simulink model "ACS_AP"  (R2022b)
settings: Solver=ode1  StartTime=0.0  StopTime=200  FixedStep=0.05  RelTol=1e-3  EnableMultiTasking=on
undefined symbols (not defined in the file): ACSP
settings Model: Creator=jmbianni  LastModifiedBy=bendr
settings SolverCC: AlgebraicLoopSolver=TrustRegion
settings DataIOCC: InitialState=[]  LimitDataPoints=on  LoadInitialState=on  SaveFormat=Array  ReturnWorkspaceOutputs=off
settings OptimizationCC: DefaultParameterBehavior=Inlined  BufferReuse=off  ExpressionDepthLimit=2147483647  LifeSpan=inf
settings DebuggingCC: ArtificialAlgebraicLoopMsg=none  UnderspecifiedInitializationDetection=Classic  MergeDetectMultiDrivingBlocksExec=none  UnconnectedInputMsg=warning  UnconnectedOutputMsg=warning  UnconnectedLineMsg=warning  StateNameClashWarn=warning  InitInArrayFormatMsg=none  SFUnexpectedBacktrackingDiag=warning  SFNoUnconditionalDefaultTransitionDiag=warning  SFExecutionAtInitializationDiag=none  SFMachineParentedDataDiag=warning  ArithmeticOperatorsInVariantConditions=warning
settings HardwareCC: ProdBitPerPointer=32  ProdBitPerSizeT=32  ProdBitPerPtrDiffT=32  ProdLargestAtomicFloat=None  ProdIntDivRoundTo=Undefined  ProdEndianess=Unspecified  ProdWordSize=32  ProdHWDeviceType=32-bit Generic
settings ModelReferenceCC: PropagateSignalLabelsOutOfModel=off
settings SFSimCC: SimUseLocalCustomCode=off  CustomCodeUndefinedFunction=UseInterfaceOnly
settings RTWCC: RTWUseLocalCustomCode=off
settings CodeAppCC: StateflowObjectComments=on
settings GRTTargetCC: TargetLangStandard=C89/C90 (ANSI)
settings ConfigComp: CovMetricSettings=dw  CovSaveCumulativeToWorkspaceVar=on  CovSaveSingleToWorkspaceVar=on  CovExternalEMLEnable=off

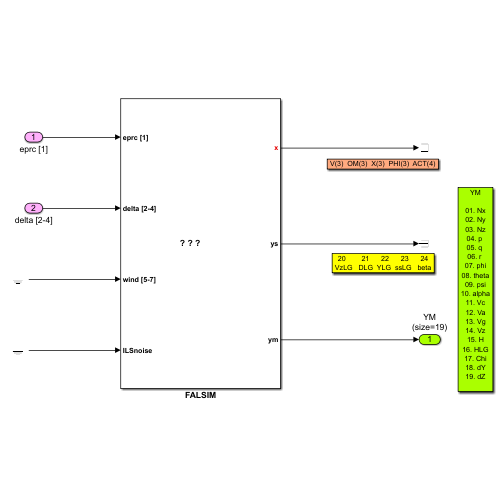
[thumbnail: Simulink's stored preview of the top-level diagram]
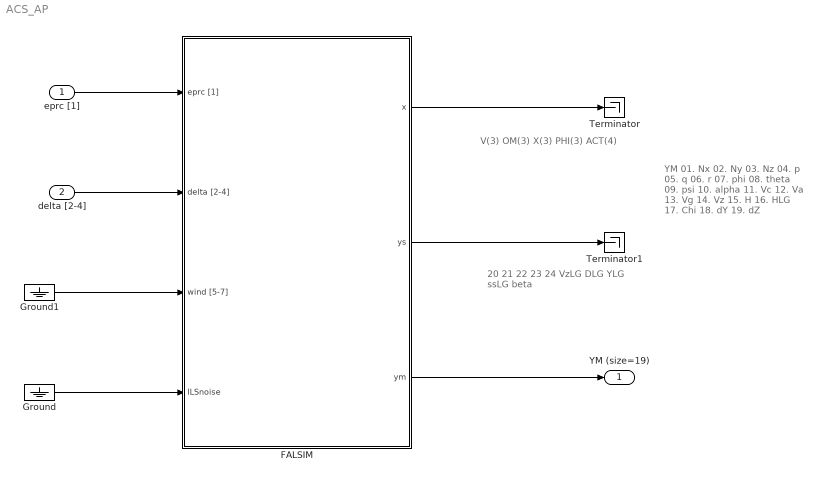
== system ACS_AP ==
  note: 20        21      22      23      24
      | VzLG   DLG  YLG  ssLG   beta
  note: YM
      |
      | 01. Nx
      | 02. Ny
      | 03. Nz
      | 04. p
      | 05. q
      | 06. r
      | 07. phi
      | 08. theta
      | 09. psi
      | 10. alpha
      | 11. Vc
      | 12. Va
      | 13. Vg
      | 14. Vz
      | 15. H
      | 16. HLG
      | 17. Chi
      | 18. dY
      | 19. dZ
  note: V(3) OM(3) X(3) PHI(3) ACT(4)
  eprc [1] : Inport
  delta [2-4] : Inport  Port=2  PortDimensions=3
  FALSIM : Subsystem
      mask Display:
      | image(imread('FALSIM.png'));
      | color('white');
      | 
      | color('red');
      | disp('http://w3.onera.fr/smac/ \n\n\n\n');
      | 
      | 
      | 
      | color('red');
      | %disp('{\bf\fontsize{12}SMAC TOOLS}', 'texmode','on');
      | 
      | color('yellow');
      | 
      | port_label('output', 1,'{\bf\fontsize{12}States}', 'texmode','on');
      | port_label('output', 2,'{\bf\fontsize{12}Non Measured Outputs}', 'texmode','on');
      | port_label('output', 3,'{\bf\fontsize{12}Measured Outputs}', 'texmode','on');
      | port_label('input', 1,'{\bf\fontsize{12}\delta_{TH}}', 'texmode','on');
      | port_label('input', 2,'{\bf\fontsize{12}\delta_A , \delta_E , \delta_R}', 'texmode','on');
      | port_label('input', 3,'{\bf\fontsize{12}W_x , W_y , W_z}', 'texmode','on');
      | port_label('input', 4,'{\bf\fontsize{12}W_{LOC} , W_{GLD}}', 'texmode','on');
  Ground : Ground
  Ground1 : Ground
  Terminator : Terminator
  Terminator1 : Terminator
  YM (size=19) : Outport
  wires:
  FALSIM/1(x) -> Terminator/1
  eprc [1]/1 -> FALSIM/1(eprc [1])
  delta [2-4]/1 -> FALSIM/2(delta [2-4])
  FALSIM/2(ys) -> Terminator1/1
  Ground/1 -> FALSIM/4(ILSnoise)
  Ground1/1 -> FALSIM/3(wind [5-7])
  FALSIM/3(ym) -> YM (size=19)/1

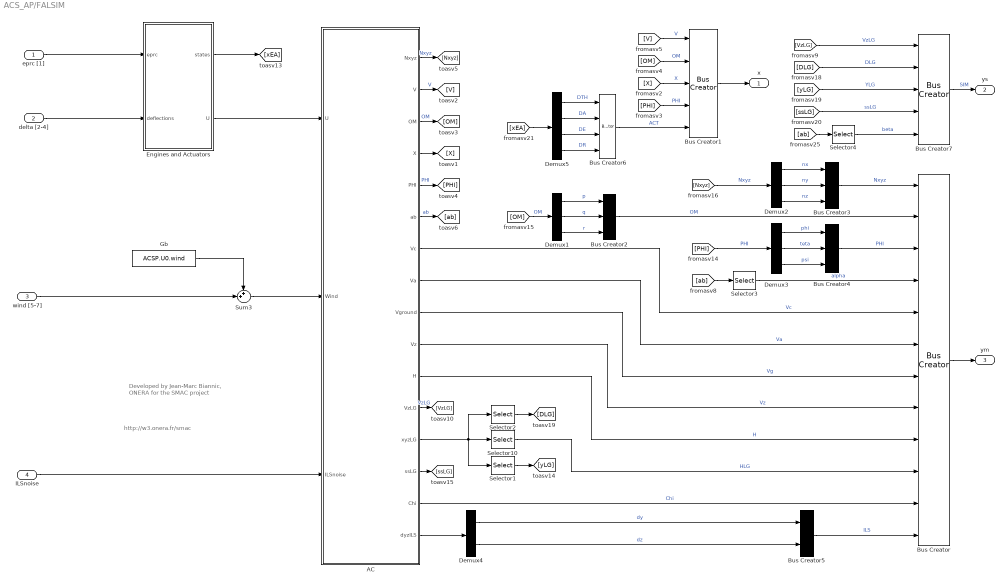
== system ACS_AP/FALSIM ==
  note: Developed by
      | Jean-Marc Biannic, ONERA
      | for the SMAC project
  note: http://w3.onera.fr/smac
  eprc [1] : Inport
  delta [2-4] : Inport  Port=2  PortDimensions=3
  wind [5-7] : Inport  Port=3  PortDimensions=3
  ILSnoise : Inport  Port=4  PortDimensions=2
  AC : Subsystem
  Bus Creator : BusCreator  Inputs=12
  Bus Creator1 : BusCreator  Inputs=5
  Bus Creator2 : BusCreator  Inputs=3
  Bus Creator3 : BusCreator  Inputs=3
  Bus Creator4 : BusCreator  Inputs=3
  Bus Creator5 : BusCreator  Inputs=2
  Bus Creator6 : BusCreator  Inputs=4
  Bus Creator7 : BusCreator  Inputs=5
  Demux1 : Demux  Outputs=3
  Demux2 : Demux  Outputs=3
  Demux3 : Demux  Outputs=3
  Demux4 : Demux  Outputs=2
  Demux5 : Demux
  Engines and Actuators : Subsystem
  Gb : Constant  Value=ACSP.U0.wind
  Selector1 : Selector  InputPortWidth=3  IndexOptions=Index vector (dialog)  Indices=2  OutputSizes=1
  Selector10 : Selector  InputPortWidth=3  IndexOptions=Index vector (dialog)  Indices=3  OutputSizes=1
  Selector2 : Selector  InputPortWidth=3  IndexOptions=Index vector (dialog)  Indices=1  OutputSizes=1
  Selector3 : Selector  InputPortWidth=2  IndexOptions=Index vector (dialog)  Indices=1  OutputSizes=1
  Selector4 : Selector  InputPortWidth=2  IndexOptions=Index vector (dialog)  Indices=2  OutputSizes=1
  Sum3 : Sum  Inputs=++|
  x : Outport
  ys : Outport  Port=2
  ym : Outport  Port=3
  wires:
  wind [5-7]/1 -> Sum3/2
  Selector3/1 -> Bus Creator/4  "alpha"
  [ab] -> Selector3/1
  Bus Creator2/1 -> Bus Creator/2  "OM"
  Demux1/3 -> Bus Creator2/3  "r"
  Demux1/2 -> Bus Creator2/2  "q"
  Demux1/1 -> Bus Creator2/1  "p"
  [OM] -> Demux1/1  "OM"
  Demux2/3 -> Bus Creator3/3  "nz"
  Demux2/2 -> Bus Creator3/2  "ny"
  Demux2/1 -> Bus Creator3/1  "nx"
  [Nxyz] -> Demux2/1  "Nxyz"
  Bus Creator3/1 -> Bus Creator/1  "Nxyz"
  Demux3/3 -> Bus Creator4/3  "psi"
  Demux3/2 -> Bus Creator4/2  "teta"
  Demux3/1 -> Bus Creator4/1  "phi"
  [PHI] -> Demux3/1  "PHI"
  Bus Creator4/1 -> Bus Creator/3  "PHI"
  AC/13(xyzLG) -> Selector1/1, Selector10/1, Selector2/1
  Selector1/1 -> [yLG]
  AC/14(ssLG) -> [ssLG]
  AC/16(dyzILS) -> Demux4/1
  Demux4/1 -> Bus Creator5/1  "dy"
  Demux4/2 -> Bus Creator5/2  "dz"
  Selector2/1 -> [DLG]
  Selector10/1 -> Bus Creator/10  "HLG"
  AC/1(Nxyz) -> [Nxyz]  "Nxyz"
  AC/2(V) -> [V]  "V"
  AC/3(OM) -> [OM]  "OM"
  AC/4(X) -> [X]
  AC/5(PHI) -> [PHI]  "PHI"
  AC/6(ab) -> [ab]  "ab"
  AC/7(Vc) -> Bus Creator/5  "Vc"
  AC/8(Va) -> Bus Creator/6  "Va"
  AC/9(Vground) -> Bus Creator/7  "Vg"
  AC/15(Chi) -> Bus Creator/11  "Chi"
  AC/12(VzLG) -> [VzLG]  "VzLG"
  [V] -> Bus Creator1/1  "V"
  [OM] -> Bus Creator1/2  "OM"
  [X] -> Bus Creator1/3  "X"
  [PHI] -> Bus Creator1/4  "PHI"
  Bus Creator1/1 -> x/1
  eprc [1]/1 -> Engines and Actuators/1(eprc)
  Engines and Actuators/2(U) -> AC/1(U)
  Engines and Actuators/1(states) -> [xEA]
  Demux5/1 -> Bus Creator6/1  "DTH"
  Demux5/2 -> Bus Creator6/2  "DA"
  Demux5/3 -> Bus Creator6/3  "DE"
  Demux5/4 -> Bus Creator6/4  "DR"
  [xEA] -> Demux5/1
  Bus Creator6/1 -> Bus Creator1/5  "ACT"
  Bus Creator5/1 -> Bus Creator/12  "ILS"
  [ab] -> Selector4/1
  AC/10(Vz) -> Bus Creator/8  "Vz"
  AC/11(H) -> Bus Creator/9  "H"
  ILSnoise/1 -> AC/3(ILSnoise)
  Gb/1 -> Sum3/1
  Sum3/1 -> AC/2(Wind)
  Bus Creator/1 -> ym/1
  Bus Creator7/1 -> ys/1  "SIM"
  delta [2-4]/1 -> Engines and Actuators/2(deflections)
  Selector4/1 -> Bus Creator7/5  "beta"
  [ssLG] -> Bus Creator7/4  "ssLG"
  [yLG] -> Bus Creator7/3  "YLG"
  [DLG] -> Bus Creator7/2  "DLG"
  [VzLG] -> Bus Creator7/1  "VzLG"

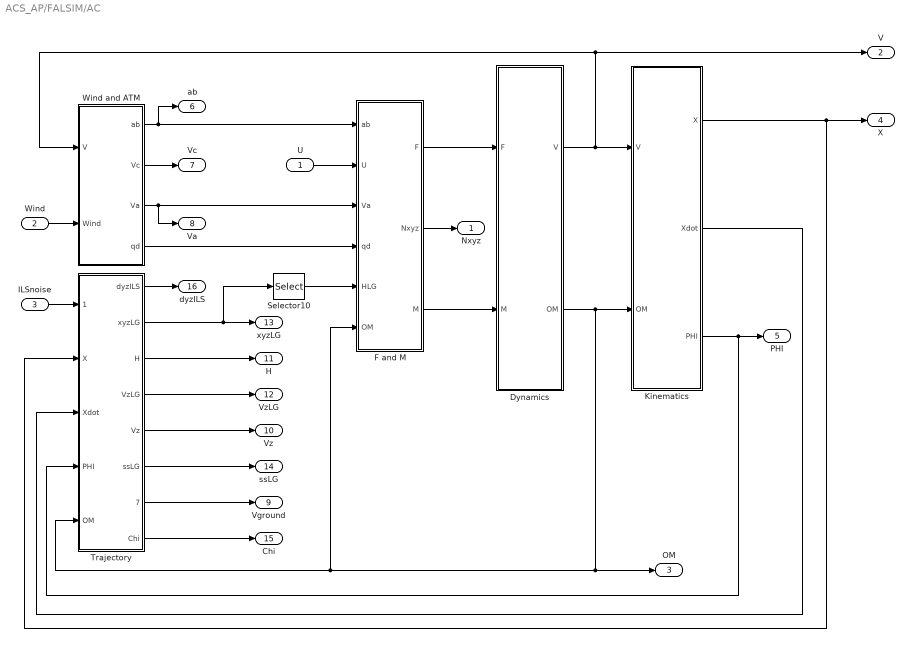
== system ACS_AP/FALSIM/AC ==
  U : Inport
  Wind : Inport  Port=2  PortDimensions=3
  ILSnoise : Inport  Port=3  PortDimensions=2
  Dynamics : Subsystem
  F and M : Subsystem
  Kinematics : Subsystem
  Selector10 : Selector  InputPortWidth=3  IndexOptions=Index vector (dialog)  Indices=3  OutputSizes=1
  Trajectory : Subsystem
  Wind and ATM : Subsystem
  Nxyz : Outport
  V : Outport  Port=2
  OM : Outport  Port=3
  X : Outport  Port=4
  PHI : Outport  Port=5
  ab : Outport  Port=6
  Vc : Outport  Port=7
  Va : Outport  Port=8
  Vground : Outport  Port=9
  Vz : Outport  Port=10
  H : Outport  Port=11
  VzLG : Outport  Port=12
  xyzLG : Outport  Port=13
  ssLG : Outport  Port=14
  Chi : Outport  Port=15
  dyzILS : Outport  Port=16
  wires:
  F and M/2(Nxyz) -> Nxyz/1
  Wind and ATM/1(ab) -> F and M/1(ab), ab/1
  U/1 -> F and M/2(U)
  Wind and ATM/4(qd) -> F and M/4(qd)
  Wind and ATM/3(Va) -> F and M/3(Va), Va/1
  Wind and ATM/2(Vc) -> Vc/1
  Wind/1 -> Wind and ATM/2(Wind)
  Kinematics/2(Xdot) -> Trajectory/3(Xdot)
  Kinematics/3(PHI) -> Trajectory/4(PHI), PHI/1
  Dynamics/2(OM) -> Kinematics/2(OM), OM/1, F and M/6(OM), Trajectory/5(OM)
  Dynamics/1(V) -> Kinematics/1(V), V/1, Wind and ATM/1(V)
  F and M/1(F) -> Dynamics/1(F)
  F and M/3(M) -> Dynamics/2(M)
  Kinematics/1(X) -> X/1, Trajectory/2(X)
  Selector10/1 -> F and M/5(HLG)
  Trajectory/2(xyzLG) -> xyzLG/1, Selector10/1
  Trajectory/1(dyzILS) -> dyzILS/1
  Trajectory/4(VzLG) -> VzLG/1
  Trajectory/8(Chi) -> Chi/1
  Trajectory/7(Vground) -> Vground/1
  Trajectory/6(ssLG) -> ssLG/1
  Trajectory/3(H) -> H/1
  Trajectory/5(Vz) -> Vz/1
  ILSnoise/1 -> Trajectory/1(ILSnoise)

== system ACS_AP/FALSIM/Engines and Actuators ==
  eprc : Inport
  deflections : Inport  Port=2
  Actuators : Subsystem
  Engines : Subsystem
  Mux : Mux  Inputs=2
  Mux1 : Mux  Inputs=2
  Sum3 : Sum  Inputs=|++
  delta0 : Constant  Value=ACSP.U0.delta
  epr0 : Constant  Value=ACSP.U0.epr
  states : Outport
  U : Outport  Port=2
  wires:
  Actuators/1(delta) -> Sum3/1, Mux1/2
  Engines/1(TH) -> Mux/1
  eprc/1 -> Engines/2(eprc)
  deflections/1 -> Actuators/1(deltac)
  epr0/1 -> Engines/1(epr0)
  Mux/1 -> U/1
  Engines/2(epr) -> Mux1/1  "EPR"
  Mux1/1 -> states/1
  Sum3/1 -> Mux/2
  delta0/1 -> Sum3/2

== system ACS_AP/FALSIM/AC/Dynamics ==
  note: F =mass*(Vdot + OM x V)
  note: M = I*OMdot + OM x (I*OM)
  F : Inport
  M : Inport  Port=2
  CP1 : Subsystem
      mask Display:
      | fprintf('CROSS \n PRODUCT');
      | color('red');
      | fprintf('\n\n');
      | fprintf(' \n \n \n z=x^y');
      | %text(3,1,'PRODUCT');
      | %text(5,1,'z=x^y');
  CP2 : Subsystem
      mask Display:
      | fprintf('CROSS \n PRODUCT');
      | color('red');
      | fprintf('\n\n');
      | fprintf(' \n \n \n z=x^y');
      | %text(3,1,'PRODUCT');
      | %text(5,1,'z=x^y');
  Inertia : Gain  Gain=reshape(ACSP.MIG.I,3,3)  Multiplication=Matrix(K*u)
  Inertia^-1 : Gain  Gain=ACSP.MIG.J  Multiplication=Matrix(K*u)
  Int_OM : Integrator  InitialCondition=ACSP.X0.OM  ContinuousStateAttributes='OM'
  Int_V : Integrator  InitialCondition=ACSP.X0.V  ContinuousStateAttributes='V'
  Mass^-1 : Gain  Gain=1/ACSP.MIG.mass
  Sum : Sum  Inputs=|+-
  Sum1 : Sum  Inputs=-+|
  V : Outport
  OM : Outport  Port=2
  wires:
  Int_V/1 -> CP2/2(y), V/1
  Sum1/1 -> Int_V/1
  Sum/1 -> Inertia^-1/1
  M/1 -> Sum/1
  Inertia^-1/1 -> Int_OM/1
  F/1 -> Mass^-1/1
  Int_OM/1 -> CP1/1(x), Inertia/1, CP2/1(x), OM/1
  CP2/1(z) -> Sum1/1
  CP1/1(z) -> Sum/2
  Mass^-1/1 -> Sum1/2
  Inertia/1 -> CP1/2(y)

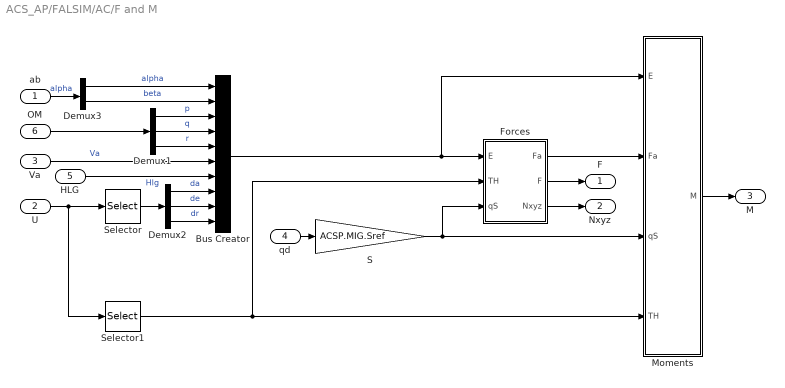
== system ACS_AP/FALSIM/AC/F and M ==
  ab : Inport
  U : Inport  Port=2
  Va : Inport  Port=3
  qd : Inport  Port=4
  HLG : Inport  Port=5
  OM : Inport  Port=6
  Bus Creator : BusCreator  Inputs=10
  Demux1 : Demux  Outputs=3
  Demux2 : Demux  Outputs=3
  Demux3 : Demux  Outputs=2
  Forces : Subsystem
  Moments : Subsystem
  S : Gain  Gain=ACSP.MIG.Sref
  Selector : Selector  InputPortWidth=4  IndexOptions=Index vector (dialog)  Indices=[2 3 4]  OutputSizes=1
  Selector1 : Selector  InputPortWidth=4  IndexOptions=Index vector (dialog)  Indices=[1]  OutputSizes=1
  F : Outport
  Nxyz : Outport  Port=2
  M : Outport  Port=3
  wires:
  Forces/3(Nxyz) -> Nxyz/1
  Selector1/1 -> Moments/4(TH), Forces/2(TH)
  Forces/2(F) -> F/1
  S/1 -> Moments/3(qS), Forces/3(qS)
  Forces/1(Fa) -> Moments/2(Fa)
  U/1 -> Selector/1, Selector1/1
  Selector/1 -> Demux2/1
  Moments/1(M) -> M/1
  Bus Creator/1 -> Moments/1(E), Forces/1(E)
  Demux1/1 -> Bus Creator/3  "p"
  Demux1/2 -> Bus Creator/4  "q"
  Demux1/3 -> Bus Creator/5  "r"
  Demux3/2 -> Bus Creator/2  "beta"
  Demux2/3 -> Bus Creator/10  "dr"
  Demux2/2 -> Bus Creator/9  "de"
  Demux2/1 -> Bus Creator/8  "da"
  Va/1 -> Bus Creator/6  "Va"
  HLG/1 -> Bus Creator/7  "Hlg"
  OM/1 -> Demux1/1
  qd/1 -> S/1
  Demux3/1 -> Bus Creator/1  "alpha"
  ab/1 -> Demux3/1  "alpha"

== system ACS_AP/FALSIM/AC/Kinematics ==
  V : Inport
  OM : Inport  Port=2
  Int_PHI : Integrator  InitialCondition=ACSP.X0.PHI  ContinuousStateAttributes='PHI'
  Int_X : Integrator  InitialCondition=ACSP.X0.X  ContinuousStateAttributes='X'
  R(PHI) : Subsystem
      mask Display:
      | fprintf('MATRIX \n PRODUCT');
      | color('red');
      | fprintf('\n\n');
      | fprintf(' \n \n \n z=M(x)*y');
  Rotations and transformations matrices : Subsystem
  T(PHI) : Subsystem
      mask Display:
      | fprintf('MATRIX \n PRODUCT');
      | color('red');
      | fprintf('\n\n');
      | fprintf(' \n \n \n z=M(x)*y');
  X : Outport
  Xdot : Outport  Port=2
  PHI : Outport  Port=3
  tag scope: RV2B=global
  wires:
  T(PHI)/1(z) -> Int_PHI/1
  Rotations and transformations matrices/2(RV2B) -> [RV2B]
  Rotations and transformations matrices/1(TPHI) -> T(PHI)/1(x)
  Rotations and transformations matrices/3(RB2V) -> R(PHI)/1(x)
  Int_X/1 -> X/1
  Int_PHI/1 -> PHI/1, Rotations and transformations matrices/1(PHI)
  R(PHI)/1(z) -> Xdot/1, Int_X/1
  V/1 -> R(PHI)/2(y)
  OM/1 -> T(PHI)/2(y)

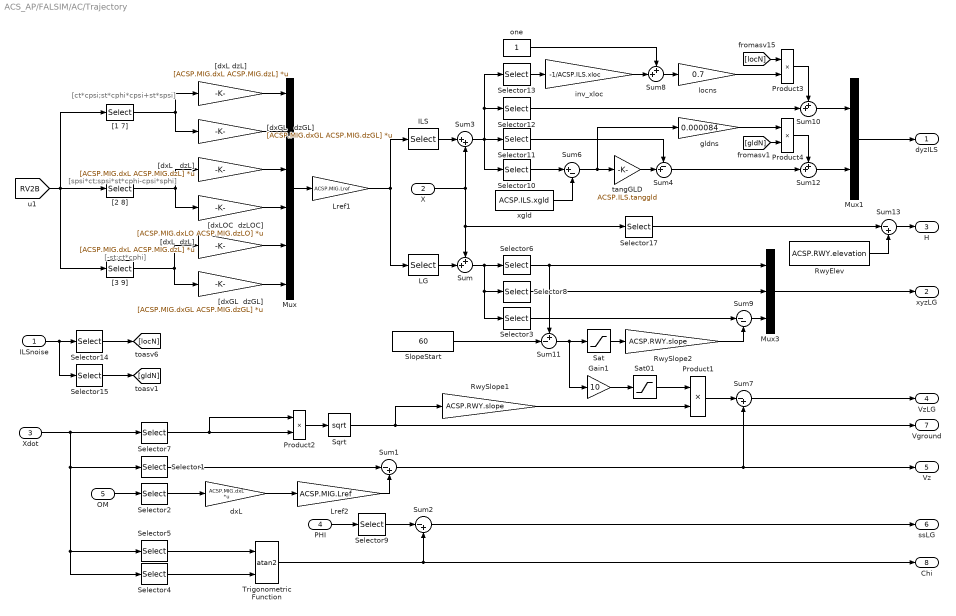
== system ACS_AP/FALSIM/AC/Trajectory ==
  note: [-st;ct*cphi]
  note: [ct*cpsi;st*cphi*cpsi+st*spsi]
  note: [spsi*ct;spsi*st*cphi-cpsi*sphi]
  ILSnoise : Inport
  X : Inport  Port=2
  Xdot : Inport  Port=3
  PHI : Inport  Port=4
  OM : Inport  Port=5
  Gain1 : Gain  Gain=10
  ILS : Selector  InputPortWidth=6  IndexOptions=Index vector (dialog)  Indices=[2 4 6]  OutputSizes=1
  LG : Selector  InputPortWidth=6  IndexOptions=Index vector (dialog)  Indices=[1 3 5]  OutputSizes=1
  Lref1 : Gain  Gain=ACSP.MIG.Lref
  Lref2 : Gain  Gain=ACSP.MIG.Lref
  Mux : Mux  Inputs=6
  Mux1 : Mux  Inputs=2
  Mux3 : Mux  Inputs=3
  Product{1..4} (4 alike) : Product  InputSameDT=on  RndMeth=Zero  SaturateOnIntegerOverflow=on  OutDataTypeStr=Inherit: Same as first input
  RwyElev : Constant  Value=ACSP.RWY.elevation
  RwySlope1 : Gain  Gain=ACSP.RWY.slope
  RwySlope2 : Gain  Gain=ACSP.RWY.slope
  Sat : Saturate  UpperLimit=1000  LowerLimit=0
  Sat01 : Saturate  UpperLimit=1  LowerLimit=0
  Selector{1,3,9,11,17} (5 alike) : Selector  InputPortWidth=3  IndexOptions=Index vector (dialog)  Indices=3  OutputSizes=1
  Selector{4,6..7,10,13} (5 alike) : Selector  InputPortWidth=3  IndexOptions=Index vector (dialog)  Indices=1  OutputSizes=1
  Selector{2,5,8,12} (4 alike) : Selector  InputPortWidth=3  IndexOptions=Index vector (dialog)  Indices=2  OutputSizes=1
  Selector14 : Selector  InputPortWidth=2  IndexOptions=Index vector (dialog)  Indices=1  OutputSizes=1
  Selector15 : Selector  InputPortWidth=2  IndexOptions=Index vector (dialog)  Indices=2  OutputSizes=1
  SlopeStart : Constant  Value=60
  Sqrt : Sqrt
  Sum{,8,10,12} (4 alike) : Sum  Inputs=++|
  Sum{1..2,7,13} (4 alike) : Sum  Inputs=|-+
  Sum11 : Sum  Inputs=+-|
  Sum3 : Sum  Inputs=|++
  Sum4 : Sum  Inputs=-+|
  Sum6 : Sum  Inputs=|+-
  Sum9 : Sum  Inputs=|--
  Trigonometric Function : Trigonometry  Operator=atan2
  "[1 7]" : Selector  InputPortWidth=9  IndexOptions=Index vector (dialog)  Indices=[1 7]  OutputSizes=1
  "[2 8]" : Selector  InputPortWidth=9  IndexOptions=Index vector (dialog)  Indices=[2 8]  OutputSizes=1
  "[3 9]" : Selector  InputPortWidth=9  IndexOptions=Index vector (dialog)  Indices=[3 9]  OutputSizes=1
  "[dxGL   dzGL]" : Gain  Gain=[ACSP.MIG.dxGL ACSP.MIG.dzGL]  Multiplication=Matrix(K*u)
  "[dxGL  dzGL]" : Gain  Gain=[ACSP.MIG.dxGL ACSP.MIG.dzGL]  Multiplication=Matrix(K*u)
  "[dxL   dzL]" : Gain  Gain=[ACSP.MIG.dxL ACSP.MIG.dzL]  Multiplication=Matrix(K*u)
  "[dxL  dzL]" : Gain  Gain=[ACSP.MIG.dxL ACSP.MIG.dzL]  Multiplication=Matrix(K*u)
  "[dxL dzL]" : Gain  Gain=[ACSP.MIG.dxL ACSP.MIG.dzL]  Multiplication=Matrix(K*u)
  "[dxLOC  dzLOC]" : Gain  Gain=[ACSP.MIG.dxLO ACSP.MIG.dzLO]  Multiplication=Matrix(K*u)
  dxL : Gain  Gain=ACSP.MIG.dxL  Multiplication=Matrix(K*u)
  gldns : Gain  Gain=0.000084
  inv_xloc : Gain  Gain=-1/ACSP.ILS.xloc
  locns : Gain  Gain=0.7
  one : Constant
  tangGLD : Gain  Gain=ACSP.ILS.tanggld
  xgld : Constant  Value=ACSP.ILS.xgld
  dyzILS : Outport
  xyzLG : Outport  Port=2
  H : Outport  Port=3
  VzLG : Outport  Port=4
  Vz : Outport  Port=5
  ssLG : Outport  Port=6
  Vground : Outport  Port=7
  Chi : Outport  Port=8
  wires:
  Xdot/1 -> Selector1/1, Selector4/1, Selector5/1, Selector7/1
  OM/1 -> Selector2/1
  Selector2/1 -> dxL/1
  dxL/1 -> Lref2/1
  Lref2/1 -> Sum1/2
  Sum1/1 -> Vz/1, Sum7/2
  [RV2B] -> "[1 7]"/1, "[3 9]"/1, "[2 8]"/1
  Selector1/1 -> Sum1/1
  Selector5/1 -> Trigonometric Function/1
  Trigonometric Function/1 -> Sum2/2, Chi/1
  "[1 7]"/1 -> "[dxL dzL]"/1, "[dxGL   dzGL]"/1
  Product2/1 -> Sqrt/1
  Selector4/1 -> Trigonometric Function/2
  Selector7/1 -> Product2/2, Product2/1
  Sqrt/1 -> Vground/1, RwySlope1/1
  "[2 8]"/1 -> "[dxL   dzL]"/1, "[dxLOC  dzLOC]"/1
  PHI/1 -> Selector9/1
  Selector9/1 -> Sum2/1
  Sum2/1 -> ssLG/1
  "[3 9]"/1 -> "[dxL  dzL]"/1, "[dxGL  dzGL]"/1
  "[dxL dzL]"/1 -> Mux/1
  "[dxGL   dzGL]"/1 -> Mux/2
  "[dxL   dzL]"/1 -> Mux/3
  "[dxLOC  dzLOC]"/1 -> Mux/4
  "[dxL  dzL]"/1 -> Mux/5
  "[dxGL  dzGL]"/1 -> Mux/6
  Mux/1 -> Lref1/1
  Lref1/1 -> LG/1, ILS/1
  ILS/1 -> Sum3/1
  Sum3/1 -> Selector10/1, Selector11/1, Selector12/1, Selector13/1
  Sum6/1 -> gldns/1, tangGLD/1
  Selector10/1 -> Sum6/1
  xgld/1 -> Sum6/2
  Mux1/1 -> dyzILS/1
  Selector12/1 -> Sum10/2
  Selector11/1 -> Sum4/1
  tangGLD/1 -> Sum4/2
  Sum4/1 -> Sum12/2
  LG/1 -> Sum/2
  X/1 -> Selector17/1, Sum/1, Sum3/2
  Sum/1 -> Selector6/1, Selector3/1, Selector8/1
  Sat01/1 -> Product1/1
  RwySlope1/1 -> Product1/2
  Sum11/1 -> Gain1/1, Sat/1
  Product1/1 -> Sum7/1
  Sat/1 -> RwySlope2/1
  Mux3/1 -> xyzLG/1
  Selector8/1 -> Mux3/2
  Selector6/1 -> Sum11/1, Mux3/1
  SlopeStart/1 -> Sum11/2
  Sum7/1 -> VzLG/1
  Gain1/1 -> Sat01/1
  Selector13/1 -> inv_xloc/1
  inv_xloc/1 -> Sum8/2
  one/1 -> Sum8/1
  Sum8/1 -> locns/1
  Sum10/1 -> Mux1/1
  locns/1 -> Product3/2
  Product3/1 -> Sum10/1
  Sum12/1 -> Mux1/2
  Product4/1 -> Sum12/1
  gldns/1 -> Product4/1
  ILSnoise/1 -> Selector15/1, Selector14/1
  Selector14/1 -> [locN]
  Selector15/1 -> [gldN]
  [locN] -> Product3/1
  [gldN] -> Product4/2
  RwyElev/1 -> Sum13/2
  Sum13/1 -> H/1
  Selector17/1 -> Sum13/1
  Sum9/1 -> Mux3/3
  RwySlope2/1 -> Sum9/2
  Selector3/1 -> Sum9/1

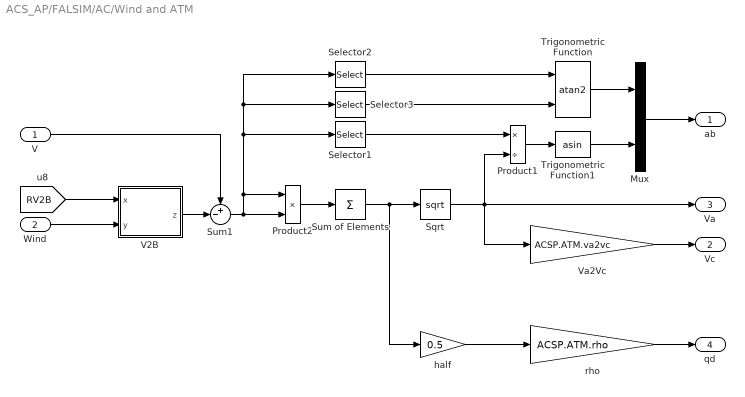
== system ACS_AP/FALSIM/AC/Wind and ATM ==
  V : Inport
  Wind : Inport  Port=2
  Mux : Mux  Inputs=2
  Product1 : Product  Inputs=*/  InputSameDT=on  RndMeth=Zero  SaturateOnIntegerOverflow=on  OutDataTypeStr=Inherit: Same as first input
  Product2 : Product  InputSameDT=on  RndMeth=Zero  SaturateOnIntegerOverflow=on  OutDataTypeStr=Inherit: Same as first input
  Selector1 : Selector  InputPortWidth=3  IndexOptions=Index vector (dialog)  Indices=2  OutputSizes=1
  Selector2 : Selector  InputPortWidth=3  IndexOptions=Index vector (dialog)  Indices=3  OutputSizes=1
  Selector3 : Selector  InputPortWidth=3  IndexOptions=Index vector (dialog)  Indices=1  OutputSizes=1
  Sqrt : Sqrt
  Sum of Elements : Sum  Inputs=+
  Sum1 : Sum  Inputs=+-|
  Trigonometric Function : Trigonometry  Operator=atan2
  Trigonometric Function1 : Trigonometry  Operator=asin
  V2B : Subsystem
      mask Display:
      | fprintf('MATRIX \n PRODUCT');
      | color('red');
      | fprintf('\n\n');
      | fprintf(' \n \n \n z=M(x)*y');
  Va2Vc : Gain  Gain=ACSP.ATM.va2vc
  half : Gain  Gain=0.5  SaturateOnIntegerOverflow=on  OutDataTypeStr=Inherit: Same as input  ParamDataTypeStr=Inherit: Same as input
  rho : Gain  Gain=ACSP.ATM.rho
  ab : Outport
  Vc : Outport  Port=2
  Va : Outport  Port=3
  qd : Outport  Port=4
  wires:
  Wind/1 -> V2B/2(y)
  rho/1 -> qd/1
  half/1 -> rho/1
  Va2Vc/1 -> Vc/1
  Sum1/1 -> Product2/2, Product2/1, Selector3/1, Selector2/1, Selector1/1
  Selector1/1 -> Product1/1
  Selector2/1 -> Trigonometric Function/1
  Selector3/1 -> Trigonometric Function/2
  [RV2B] -> V2B/1(x)
  V2B/1(z) -> Sum1/2
  V/1 -> Sum1/1
  Product2/1 -> Sum of Elements/1
  Sqrt/1 -> Va/1, Product1/2, Va2Vc/1
  Product1/1 -> Trigonometric Function1/1
  Sum of Elements/1 -> Sqrt/1, half/1
  Trigonometric Function/1 -> Mux/1
  Trigonometric Function1/1 -> Mux/2
  Mux/1 -> ab/1

== system ACS_AP/FALSIM/Engines and Actuators/Actuators ==
  deltac : Inport
  Gain2 : Gain  Gain=1./ACSP.ACT.tau
  Int_ASD : Integrator  ContinuousStateAttributes='xASD'
  ML [55 25 30] : Saturate  UpperLimit=ACSP.ACT.ML  LowerLimit=-ACSP.ACT.ML
  RL [60 20 30] : Saturate  UpperLimit=ACSP.ACT.RL  LowerLimit=-ACSP.ACT.RL
  Sum : Sum  Inputs=|+-
  delta : Outport
  wires:
  ML [55 25 30]/1 -> delta/1
  Sum/1 -> Gain2/1
  deltac/1 -> Sum/1
  Int_ASD/1 -> ML [55 25 30]/1, Sum/2
  RL [60 20 30]/1 -> Int_ASD/1
  Gain2/1 -> RL [60 20 30]/1

== system ACS_AP/FALSIM/Engines and Actuators/Engines ==
  epr0 : Inport
  eprc : Inport  Port=2
  EML : Saturate  UpperLimit=ACSP.ENG.UML  LowerLimit=ACSP.ENG.LML
  ERL : Saturate  UpperLimit=ACSP.ENG.RL  LowerLimit=-ACSP.ENG.RL
  Gain1 : Gain  Gain=1/ACSP.ENG.tau
  Gain2 : Gain  Gain=ACSP.ENG.Ga
  Gb : Constant  Value=ACSP.ENG.Gb
  Int_ENG : Integrator  ContinuousStateAttributes='xENG'
  Sum : Sum  Inputs=|+-
  Sum1 : Sum  Inputs=+-|
  Sum2 : Sum  Inputs=|++
  Sum3 : Sum  Inputs=++|
  TH : Outport
  epr : Outport  Port=2
  wires:
  Sum2/1 -> EML/1
  Gb/1 -> Sum3/1
  Gain2/1 -> Sum3/2
  Sum3/1 -> TH/1
  eprc/1 -> Sum/1
  Int_ENG/1 -> Sum2/1, Sum/2
  ERL/1 -> Int_ENG/1
  Gain1/1 -> ERL/1
  Sum/1 -> Gain1/1
  EML/1 -> Sum1/1, Gain2/1
  epr0/1 -> Sum1/2, Sum2/2
  Sum1/1 -> epr/1

== system ACS_AP/FALSIM/AC/Dynamics/CP1 ==
  x : Inport
  y : Inport  Port=2
  Mux : Mux  Inputs=2
  Mux1 : Mux  Inputs=3
  Y1 : Fcn  Expr=u(2)*u(6)-u(3)*u(5)
  Y2 : Fcn  Expr=u(3)*u(4)-u(1)*u(6)
  Y3 : Fcn  Expr=u(1)*u(5)-u(2)*u(4)
  z : Outport
  wires:
  Mux1/1 -> z/1
  Y2/1 -> Mux1/2
  Y1/1 -> Mux1/1
  Y3/1 -> Mux1/3
  y/1 -> Mux/2
  Mux/1 -> Y2/1, Y3/1, Y1/1
  x/1 -> Mux/1

== system ACS_AP/FALSIM/AC/Dynamics/CP2 ==
  x : Inport
  y : Inport  Port=2
  Mux : Mux  Inputs=2
  Mux1 : Mux  Inputs=3
  Y1 : Fcn  Expr=u(2)*u(6)-u(3)*u(5)
  Y2 : Fcn  Expr=u(3)*u(4)-u(1)*u(6)
  Y3 : Fcn  Expr=u(1)*u(5)-u(2)*u(4)
  z : Outport
  wires:
  Mux1/1 -> z/1
  Y2/1 -> Mux1/2
  Y1/1 -> Mux1/1
  Y3/1 -> Mux1/3
  y/1 -> Mux/2
  Mux/1 -> Y2/1, Y3/1, Y1/1
  x/1 -> Mux/1

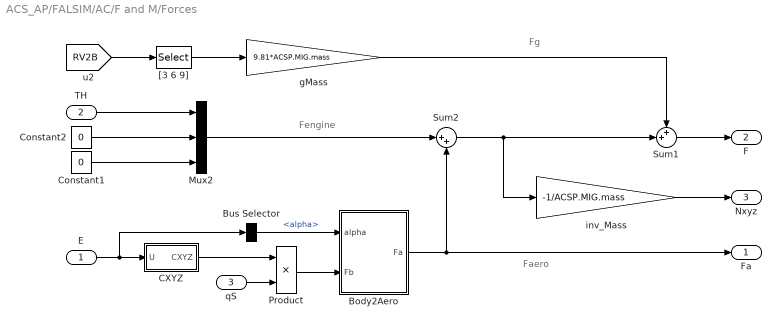
== system ACS_AP/FALSIM/AC/F and M/Forces ==
  note: Fg
  note: Fengine
  note: Faero
  E : Inport
  TH : Inport  Port=2
  qS : Inport  Port=3
  Body2Aero : Subsystem
  Bus Selector : BusSelector  OutputSignals=alpha
  CXYZ : Subsystem
  Constant1 : Constant  Value=0
  Constant2 : Constant  Value=0
  Mux2 : Mux  Inputs=3
  Product : Product  RndMeth=Zero
  Sum1 : Sum  Inputs=++|
  Sum2 : Sum  Inputs=|++
  "[3 6 9]" : Selector  InputPortWidth=9  IndexOptions=Index vector (dialog)  Indices=[3 6 9]  OutputSizes=1
  gMass : Gain  Gain=9.81*ACSP.MIG.mass
  inv_Mass : Gain  Gain=-1/ACSP.MIG.mass
  Fa : Outport
  F : Outport  Port=2
  Nxyz : Outport  Port=3
  wires:
  inv_Mass/1 -> Nxyz/1
  gMass/1 -> Sum1/1
  Sum2/1 -> Sum1/2, inv_Mass/1
  Mux2/1 -> Sum2/1
  Bus Selector/1 -> Body2Aero/1(alpha)  "<alpha>"
  CXYZ/1(CXYZ) -> Product/1
  E/1 -> CXYZ/1(U), Bus Selector/1
  Product/1 -> Body2Aero/2(Fb)
  Body2Aero/1(Fa) -> Fa/1, Sum2/2
  qS/1 -> Product/2
  Sum1/1 -> F/1
  "[3 6 9]"/1 -> gMass/1
  [RV2B] -> "[3 6 9]"/1
  Constant1/1 -> Mux2/3
  Constant2/1 -> Mux2/2
  TH/1 -> Mux2/1

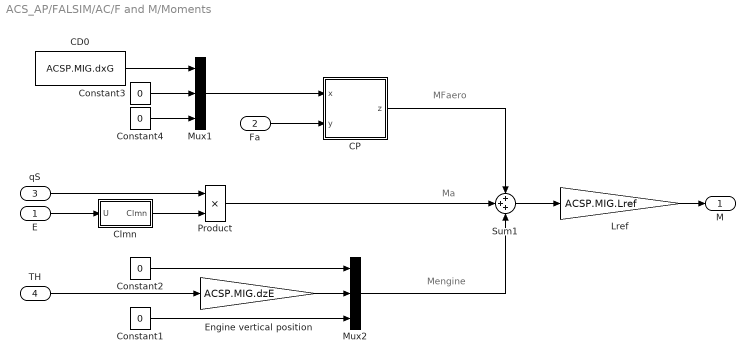
== system ACS_AP/FALSIM/AC/F and M/Moments ==
  note: Ma
  note: Mengine
  note: MFaero
  E : Inport
  Fa : Inport  Port=2
  qS : Inport  Port=3
  TH : Inport  Port=4
  CD0 : Constant  Value=ACSP.MIG.dxG
  CP : Subsystem
      mask Display:
      | fprintf('CROSS \n PRODUCT');
      | color('red');
      | fprintf('\n\n');
      | fprintf(' \n \n \n z=x^y');
      | %text(3,1,'PRODUCT');
      | %text(5,1,'z=x^y');
  Clmn : Subsystem
  Constant{1..4} (4 alike) : Constant  Value=0
  Engine vertical position : Gain  Gain=ACSP.MIG.dzE
  Lref : Gain  Gain=ACSP.MIG.Lref
  Mux1 : Mux  Inputs=3
  Mux2 : Mux  Inputs=3
  Product : Product  RndMeth=Zero
  Sum1 : Sum  Inputs=+++
  M : Outport
  wires:
  E/1 -> Clmn/1(U)
  Clmn/1(Clmn) -> Product/2
  Lref/1 -> M/1
  Mux2/1 -> Sum1/3
  Product/1 -> Sum1/2
  CD0/1 -> Mux1/1
  Constant4/1 -> Mux1/3
  Constant3/1 -> Mux1/2
  CP/1(z) -> Sum1/1
  Mux1/1 -> CP/1(x)
  Fa/1 -> CP/2(y)
  qS/1 -> Product/1
  Constant2/1 -> Mux2/1
  Engine vertical position/1 -> Mux2/2
  TH/1 -> Engine vertical position/1
  Sum1/1 -> Lref/1
  Constant1/1 -> Mux2/3

== system ACS_AP/FALSIM/AC/Kinematics/R(PHI) ==
  x : Inport
  y : Inport  Port=2
  Mux : Mux  Inputs=2
  Mux1 : Mux  Inputs=3
  Y1 : Fcn  Expr=u(1)*u(10)+u(2)*u(11)+u(3)*u(12)
  Y2 : Fcn  Expr=u(4)*u(10)+u(5)*u(11)+u(6)*u(12)
  Y3 : Fcn  Expr=u(7)*u(10)+u(8)*u(11)+u(9)*u(12)
  z : Outport
  wires:
  Mux1/1 -> z/1
  Y2/1 -> Mux1/2
  Y1/1 -> Mux1/1
  Y3/1 -> Mux1/3
  y/1 -> Mux/2
  Mux/1 -> Y2/1, Y1/1, Y3/1
  x/1 -> Mux/1

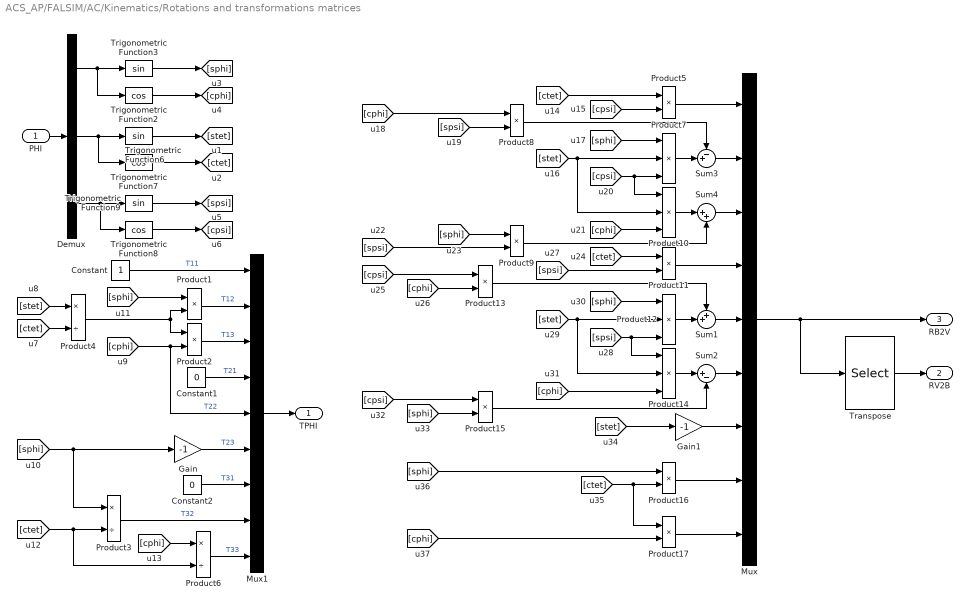
== system ACS_AP/FALSIM/AC/Kinematics/Rotations and transformations matrices ==
  PHI : Inport
  Constant : Constant
  Constant1 : Constant  Value=0
  Constant2 : Constant  Value=0
  Demux : Demux  Outputs=3
  Gain : Gain  Gain=-1
  Gain1 : Gain  Gain=-1
  Mux : Mux  Inputs=9
  Mux1 : Mux  Inputs=9
  Product{1..2,5,8..9,11,13,15..17} (10 alike) : Product  InputSameDT=on  RndMeth=Zero  SaturateOnIntegerOverflow=on  OutDataTypeStr=Inherit: Same as first input
  Product{7,10,12,14} (4 alike) : Product  Inputs=3  InputSameDT=on  RndMeth=Zero  SaturateOnIntegerOverflow=on  OutDataTypeStr=Inherit: Same as first input
  Product3 : Product  Inputs=*/  InputSameDT=on  RndMeth=Zero  SaturateOnIntegerOverflow=on  OutDataTypeStr=Inherit: Same as first input
  Product4 : Product  Inputs=*/  InputSameDT=on  RndMeth=Zero  SaturateOnIntegerOverflow=on  OutDataTypeStr=Inherit: Same as first input
  Product6 : Product  Inputs=*/  InputSameDT=on  RndMeth=Zero  SaturateOnIntegerOverflow=on  OutDataTypeStr=Inherit: Same as first input
  Sum1 : Sum  Inputs=++|
  Sum2 : Sum  Inputs=|+-
  Sum3 : Sum  Inputs=-+|
  Sum4 : Sum  Inputs=|++
  Transpose : Selector  InputPortWidth=9  IndexOptions=Index vector (dialog)  Indices=[1 4 7 2 5 8 3 6 9]  OutputSizes=1
  Trigonometric Function2 : Trigonometry  Operator=cos
  Trigonometric Function3 : Trigonometry
  Trigonometric Function6 : Trigonometry
  Trigonometric Function7 : Trigonometry  Operator=cos
  Trigonometric Function8 : Trigonometry  Operator=cos
  Trigonometric Function9 : Trigonometry
  TPHI : Outport
  RV2B : Outport  Port=2
  RB2V : Outport  Port=3
  wires:
  Transpose/1 -> RV2B/1
  Mux/1 -> RB2V/1, Transpose/1
  Mux1/1 -> TPHI/1
  [cphi] -> Product17/2
  [sphi] -> Product16/1
  Product17/1 -> Mux/9
  [ctet] -> Product16/2, Product17/1
  Product16/1 -> Mux/8
  [stet] -> Gain1/1
  Gain1/1 -> Mux/7
  Product15/1 -> Sum2/2
  [sphi] -> Product15/2
  [cpsi] -> Product15/1
  [cphi] -> Product14/3
  Sum2/1 -> Mux/6
  Product14/1 -> Sum2/1
  [sphi] -> Product12/1
  [stet] -> Product12/2, Product14/2
  [spsi] -> Product12/3, Product14/1
  [spsi] -> Product11/2
  Product13/1 -> Sum1/1
  [cphi] -> Product13/2
  [cpsi] -> Product13/1
  Sum1/1 -> Mux/5
  Product12/1 -> Sum1/2
  Product11/1 -> Mux/4
  [ctet] -> Product11/1
  [spsi] -> Product9/2
  [sphi] -> Product9/1
  Product9/1 -> Sum4/2
  [cphi] -> Product10/3
  [cpsi] -> Product7/3, Product10/1
  [sphi] -> Product7/1
  Product10/1 -> Sum4/1
  Sum4/1 -> Mux/3
  Product8/1 -> Sum3/1
  Sum3/1 -> Mux/2
  Product7/1 -> Sum3/2
  [spsi] -> Product8/2
  [cphi] -> Product8/1
  [stet] -> Product7/2, Product10/2
  [cpsi] -> Product5/2
  [ctet] -> Product5/1
  Product5/1 -> Mux/1
  PHI/1 -> Demux/1
  Product3/1 -> Mux1/8  "T32"
  [cphi] -> Product6/1
  Gain/1 -> Mux1/6  "T23"
  Constant2/1 -> Mux1/7  "T31"
  [sphi] -> Gain/1, Product3/1
  Product6/1 -> Mux1/9  "T33"
  Constant1/1 -> Mux1/4  "T21"
  Product2/1 -> Mux1/3  "T13"
  Constant/1 -> Mux1/1  "T11"
  [ctet] -> Product3/2, Product6/2
  Product1/1 -> Mux1/2  "T12"
  [cphi] -> Product2/2, Mux1/5  "T22"
  Trigonometric Function3/1 -> [sphi]
  Demux/1 -> Trigonometric Function2/1, Trigonometric Function3/1
  Trigonometric Function2/1 -> [cphi]
  Demux/2 -> Trigonometric Function6/1, Trigonometric Function7/1
  Trigonometric Function7/1 -> [ctet]
  Trigonometric Function6/1 -> [stet]
  Demux/3 -> Trigonometric Function8/1, Trigonometric Function9/1
  Trigonometric Function9/1 -> [spsi]
  Trigonometric Function8/1 -> [cpsi]
  Product4/1 -> Product2/1, Product1/2
  [sphi] -> Product1/1
  [ctet] -> Product4/2
  [stet] -> Product4/1

== system ACS_AP/FALSIM/AC/Kinematics/T(PHI) ==
  x : Inport
  y : Inport  Port=2
  Mux : Mux  Inputs=2
  Mux1 : Mux  Inputs=3
  Y1 : Fcn  Expr=u(1)*u(10)+u(2)*u(11)+u(3)*u(12)
  Y2 : Fcn  Expr=u(4)*u(10)+u(5)*u(11)+u(6)*u(12)
  Y3 : Fcn  Expr=u(7)*u(10)+u(8)*u(11)+u(9)*u(12)
  z : Outport
  wires:
  Mux1/1 -> z/1
  Y2/1 -> Mux1/2
  Y1/1 -> Mux1/1
  Y3/1 -> Mux1/3
  y/1 -> Mux/2
  Mux/1 -> Y2/1, Y1/1, Y3/1
  x/1 -> Mux/1

== system ACS_AP/FALSIM/AC/Wind and ATM/V2B ==
  x : Inport
  y : Inport  Port=2
  Mux : Mux  Inputs=2
  Mux1 : Mux  Inputs=3
  Y1 : Fcn  Expr=u(1)*u(10)+u(2)*u(11)+u(3)*u(12)
  Y2 : Fcn  Expr=u(4)*u(10)+u(5)*u(11)+u(6)*u(12)
  Y3 : Fcn  Expr=u(7)*u(10)+u(8)*u(11)+u(9)*u(12)
  z : Outport
  wires:
  Mux1/1 -> z/1
  Y2/1 -> Mux1/2
  Y1/1 -> Mux1/1
  Y3/1 -> Mux1/3
  y/1 -> Mux/2
  Mux/1 -> Y2/1, Y1/1, Y3/1
  x/1 -> Mux/1

== system ACS_AP/FALSIM/AC/F and M/Forces/Body2Aero ==
  alpha : Inport
  Fb : Inport  Port=2
  Fy : Selector  InputPortWidth=5  IndexOptions=Index vector (dialog)  Indices=4  OutputSizes=1
  Mux : Mux  Inputs=[1 1 3]
  Mux3 : Mux  Inputs=3
  Trigonometric Function1 : Trigonometry
  Trigonometric Function2 : Trigonometry  Operator=cos
  ca*Fx-sa*Fz : Fcn  Expr=u(1)*u(3)-u(2)*u(5)
  sa*Fx+ca*Fz : Fcn  Expr=u(2)*u(3)+u(1)*u(5)
  Fa : Outport
  wires:
  Fy/1 -> Mux3/2
  Mux3/1 -> Fa/1
  Mux/1 -> Fy/1, ca*Fx-sa*Fz/1, sa*Fx+ca*Fz/1
  ca*Fx-sa*Fz/1 -> Mux3/1
  sa*Fx+ca*Fz/1 -> Mux3/3
  Trigonometric Function2/1 -> Mux/1
  Trigonometric Function1/1 -> Mux/2
  Fb/1 -> Mux/3
  alpha/1 -> Trigonometric Function2/1, Trigonometric Function1/1

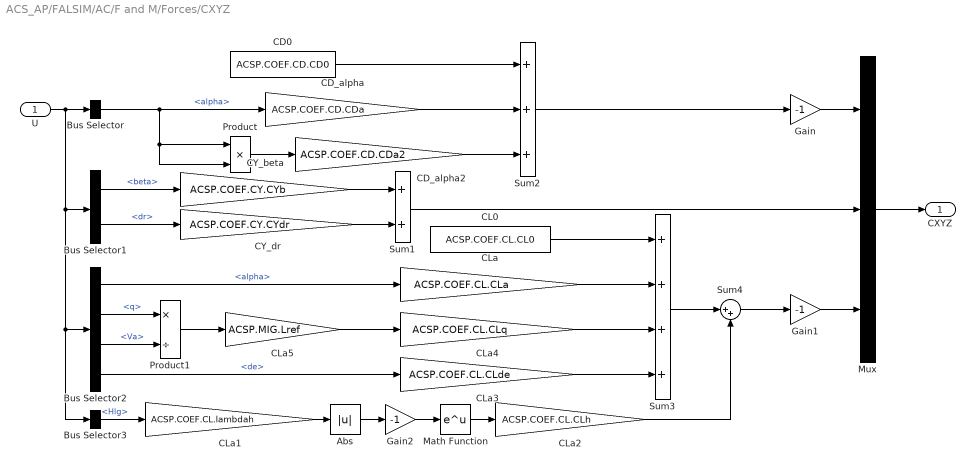
== system ACS_AP/FALSIM/AC/F and M/Forces/CXYZ ==
  U : Inport
  Abs : Abs  SaturateOnIntegerOverflow=off
  Bus Selector : BusSelector  OutputSignals=alpha
  Bus Selector1 : BusSelector  OutputSignals=beta,dr
  Bus Selector2 : BusSelector  OutputSignals=alpha,q,Va,de
  Bus Selector3 : BusSelector  OutputSignals=Hlg
  CD0 : Constant  Value=ACSP.COEF.CD.CD0
  CD_alpha : Gain  Gain=ACSP.COEF.CD.CDa
  CD_alpha2 : Gain  Gain=ACSP.COEF.CD.CDa2
  CL0 : Constant  Value=ACSP.COEF.CL.CL0
  CLa : Gain  Gain=ACSP.COEF.CL.CLa
  CLa1 : Gain  Gain=ACSP.COEF.CL.lambdah
  CLa2 : Gain  Gain=ACSP.COEF.CL.CLh
  CLa3 : Gain  Gain=ACSP.COEF.CL.CLde
  CLa4 : Gain  Gain=ACSP.COEF.CL.CLq
  CLa5 : Gain  Gain=ACSP.MIG.Lref
  CY_beta : Gain  Gain=ACSP.COEF.CY.CYb
  CY_dr : Gain  Gain=ACSP.COEF.CY.CYdr
  Gain : Gain  Gain=-1
  Gain1 : Gain  Gain=-1
  Gain2 : Gain  Gain=-1
  Math Function : Math  SignedPower=on
  Mux : Mux  Inputs=3
  Product : Product  RndMeth=Zero
  Product1 : Product  Inputs=*/  RndMeth=Zero
  Sum1 : Sum
  Sum2 : Sum  Inputs=+++
  Sum3 : Sum  Inputs=++++
  Sum4 : Sum  Inputs=|++
  CXYZ : Outport
  wires:
  Sum4/1 -> Gain1/1
  Sum2/1 -> Gain/1
  CLa4/1 -> Sum3/3
  CLa2/1 -> Sum4/2
  Bus Selector3/1 -> CLa1/1  "<Hlg>"
  Sum3/1 -> Sum4/1
  CLa3/1 -> Sum3/4
  Bus Selector2/4 -> CLa3/1  "<de>"
  Mux/1 -> CXYZ/1
  Sum1/1 -> Mux/2
  Gain/1 -> Mux/1
  Gain1/1 -> Mux/3
  CL0/1 -> Sum3/1
  Bus Selector2/1 -> CLa/1  "<alpha>"
  Bus Selector2/3 -> Product1/2  "<Va>"
  Bus Selector2/2 -> Product1/1  "<q>"
  CLa/1 -> Sum3/2
  Product1/1 -> CLa5/1
  Math Function/1 -> CLa2/1
  Abs/1 -> Gain2/1
  Gain2/1 -> Math Function/1
  CLa1/1 -> Abs/1
  CD0/1 -> Sum2/1
  CD_alpha2/1 -> Sum2/3
  CD_alpha/1 -> Sum2/2
  CY_dr/1 -> Sum1/2
  CY_beta/1 -> Sum1/1
  Bus Selector1/2 -> CY_dr/1  "<dr>"
  Bus Selector1/1 -> CY_beta/1  "<beta>"
  Product/1 -> CD_alpha2/1
  Bus Selector/1 -> CD_alpha/1, Product/1, Product/2  "<alpha>"
  U/1 -> Bus Selector/1, Bus Selector1/1, Bus Selector2/1, Bus Selector3/1
  CLa5/1 -> CLa4/1

== system ACS_AP/FALSIM/AC/F and M/Moments/CP ==
  x : Inport
  y : Inport  Port=2
  Mux : Mux  Inputs=2
  Mux1 : Mux  Inputs=3
  Y1 : Fcn  Expr=u(2)*u(6)-u(3)*u(5)
  Y2 : Fcn  Expr=u(3)*u(4)-u(1)*u(6)
  Y3 : Fcn  Expr=u(1)*u(5)-u(2)*u(4)
  z : Outport
  wires:
  Mux1/1 -> z/1
  Y2/1 -> Mux1/2
  Y1/1 -> Mux1/1
  Y3/1 -> Mux1/3
  y/1 -> Mux/2
  Mux/1 -> Y2/1, Y3/1, Y1/1
  x/1 -> Mux/1

== system ACS_AP/FALSIM/AC/F and M/Moments/Clmn ==
  U : Inport
  Cl : Subsystem
  Cm : Subsystem
  Cn : Subsystem
  Mux : Mux  Inputs=3
  Clmn : Outport
  wires:
  Mux/1 -> Clmn/1
  Cn/1(Cn) -> Mux/3
  Cm/1(Cm) -> Mux/2
  Cl/1(Cl) -> Mux/1
  U/1 -> Cm/1(U), Cl/1(U), Cn/1(U)

== system ACS_AP/FALSIM/AC/F and M/Moments/Clmn/Cl ==
  U : Inport
  Bus Selector : BusSelector  OutputSignals=beta,p,alpha,r,Va,da,dr
  CD0 : Constant  Value=ACSP.COEF.Cl.Clr0
  CD_alpha : Gain  Gain=ACSP.COEF.Cl.Clb
  CD_alpha1 : Gain  Gain=ACSP.COEF.Cl.Clp
  CD_alpha2 : Gain  Gain=ACSP.COEF.Cl.Clra
  CD_alpha3 : Gain  Gain=ACSP.COEF.Cl.Clda
  CD_alpha4 : Gain  Gain=ACSP.COEF.Cl.Cldr
  CLa3 : Gain  Gain=ACSP.MIG.Lref
  Product1 : Product  RndMeth=Zero
  Product2 : Product  Inputs=*/  RndMeth=Zero
  Sum1 : Sum
  Sum2 : Sum  Inputs=+++
  Sum4 : Sum  Inputs=|++
  Sum5 : Sum  Inputs=++|
  Cl : Outport
  wires:
  CD0/1 -> Sum4/2
  Sum5/1 -> Product2/1
  CLa3/1 -> Sum2/2
  Sum1/1 -> Sum2/3
  Bus Selector/5 -> Product2/2  "<Va>"
  Bus Selector/2 -> CD_alpha1/1  "<p>"
  Sum2/1 -> Cl/1
  CD_alpha4/1 -> Sum1/2
  CD_alpha2/1 -> Sum4/1
  Bus Selector/1 -> CD_alpha/1  "<beta>"
  CD_alpha3/1 -> Sum1/1
  CD_alpha/1 -> Sum2/1
  Sum4/1 -> Product1/1
  Product2/1 -> CLa3/1
  Bus Selector/7 -> CD_alpha4/1  "<dr>"
  CD_alpha1/1 -> Sum5/1
  Product1/1 -> Sum5/2
  Bus Selector/6 -> CD_alpha3/1  "<da>"
  Bus Selector/4 -> Product1/2  "<r>"
  Bus Selector/3 -> CD_alpha2/1  "<alpha>"
  U/1 -> Bus Selector/1

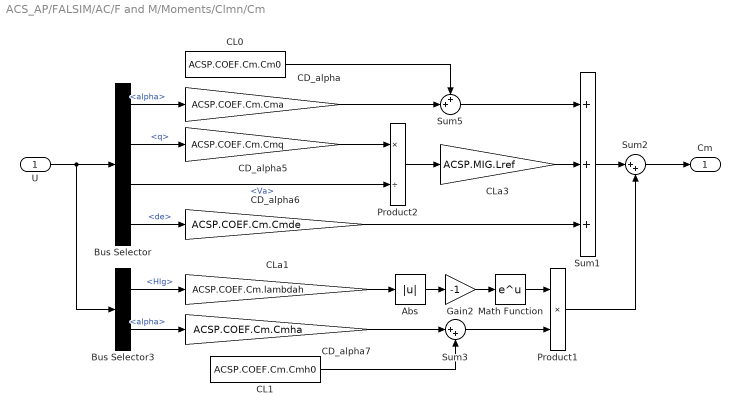
== system ACS_AP/FALSIM/AC/F and M/Moments/Clmn/Cm ==
  U : Inport
  Abs : Abs  SaturateOnIntegerOverflow=off
  Bus Selector : BusSelector  OutputSignals=alpha,q,Va,de
  Bus Selector3 : BusSelector  OutputSignals=Hlg,alpha
  CD_alpha : Gain  Gain=ACSP.COEF.Cm.Cma
  CD_alpha5 : Gain  Gain=ACSP.COEF.Cm.Cmq
  CD_alpha6 : Gain  Gain=ACSP.COEF.Cm.Cmde
  CD_alpha7 : Gain  Gain=ACSP.COEF.Cm.Cmha
  CL0 : Constant  Value=ACSP.COEF.Cm.Cm0
  CL1 : Constant  Value=ACSP.COEF.Cm.Cmh0
  CLa1 : Gain  Gain=ACSP.COEF.Cm.lambdah
  CLa3 : Gain  Gain=ACSP.MIG.Lref
  Gain2 : Gain  Gain=-1
  Math Function : Math  SignedPower=on
  Product1 : Product  RndMeth=Zero
  Product2 : Product  Inputs=*/  RndMeth=Zero
  Sum1 : Sum  Inputs=+++
  Sum2 : Sum  Inputs=|++
  Sum3 : Sum  Inputs=|++
  Sum5 : Sum  Inputs=++|
  Cm : Outport
  wires:
  Sum2/1 -> Cm/1
  Sum5/1 -> Sum1/1
  CLa3/1 -> Sum1/2
  CD_alpha6/1 -> Sum1/3
  CL0/1 -> Sum5/1
  CD_alpha/1 -> Sum5/2
  Sum3/1 -> Product1/2
  CL1/1 -> Sum3/2
  CD_alpha7/1 -> Sum3/1
  Bus Selector3/2 -> CD_alpha7/1  "<alpha>"
  Bus Selector3/1 -> CLa1/1  "<Hlg>"
  Math Function/1 -> Product1/1
  Product1/1 -> Sum2/2
  Sum1/1 -> Sum2/1
  Abs/1 -> Gain2/1
  Gain2/1 -> Math Function/1
  CLa1/1 -> Abs/1
  Bus Selector/4 -> CD_alpha6/1  "<de>"
  Product2/1 -> CLa3/1
  Bus Selector/3 -> Product2/2  "<Va>"
  CD_alpha5/1 -> Product2/1
  Bus Selector/2 -> CD_alpha5/1  "<q>"
  Bus Selector/1 -> CD_alpha/1  "<alpha>"
  U/1 -> Bus Selector/1, Bus Selector3/1

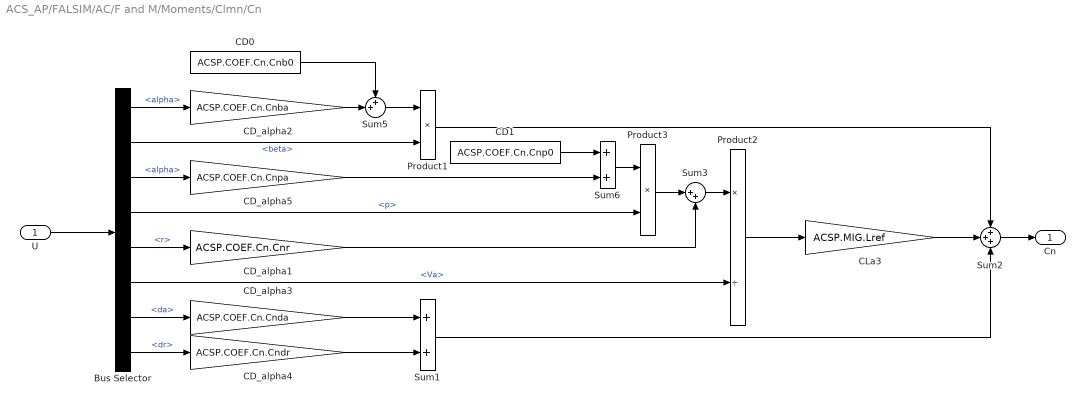
== system ACS_AP/FALSIM/AC/F and M/Moments/Clmn/Cn ==
  U : Inport
  Bus Selector : BusSelector  OutputSignals=alpha,beta,alpha,p,r,Va,da,dr
  CD0 : Constant  Value=ACSP.COEF.Cn.Cnb0
  CD1 : Constant  Value=ACSP.COEF.Cn.Cnp0
  CD_alpha1 : Gain  Gain=ACSP.COEF.Cn.Cnr
  CD_alpha2 : Gain  Gain=ACSP.COEF.Cn.Cnba
  CD_alpha3 : Gain  Gain=ACSP.COEF.Cn.Cnda
  CD_alpha4 : Gain  Gain=ACSP.COEF.Cn.Cndr
  CD_alpha5 : Gain  Gain=ACSP.COEF.Cn.Cnpa
  CLa3 : Gain  Gain=ACSP.MIG.Lref
  Product1 : Product  RndMeth=Zero
  Product2 : Product  Inputs=*/  RndMeth=Zero
  Product3 : Product  RndMeth=Zero
  Sum1 : Sum
  Sum2 : Sum  Inputs=+++
  Sum3 : Sum  Inputs=|++
  Sum5 : Sum  Inputs=++|
  Sum6 : Sum
  Cn : Outport
  wires:
  Sum3/1 -> Product2/1
  Product3/1 -> Sum3/1
  CLa3/1 -> Sum2/2
  Sum1/1 -> Sum2/3
  CD_alpha4/1 -> Sum1/2
  CD_alpha3/1 -> Sum1/1
  Bus Selector/8 -> CD_alpha4/1  "<dr>"
  Bus Selector/7 -> CD_alpha3/1  "<da>"
  Bus Selector/6 -> Product2/2  "<Va>"
  CD_alpha1/1 -> Sum3/2
  Bus Selector/5 -> CD_alpha1/1  "<r>"
  Bus Selector/4 -> Product3/2  "<p>"
  Sum6/1 -> Product3/1
  CD1/1 -> Sum6/1
  CD_alpha5/1 -> Sum6/2
  Product1/1 -> Sum2/1
  Bus Selector/3 -> CD_alpha5/1  "<alpha>"
  Sum5/1 -> Product1/1
  Bus Selector/2 -> Product1/2  "<beta>"
  CD0/1 -> Sum5/1
  CD_alpha2/1 -> Sum5/2
  Bus Selector/1 -> CD_alpha2/1  "<alpha>"
  Sum2/1 -> Cn/1
  Product2/1 -> CLa3/1
  U/1 -> Bus Selector/1
